simulink model "motorload"  (R2014b)
settings: Solver=ode23tb  StartTime=0.0  StopTime=10  MaxStep=.0001  MinStep=0.00001  RelTol=1e-3
undefined symbols (not defined in the file): sigbuilder_block
libraries: powerlib x145, simulink x25, powerlib_extras x4, dsparch4 x2, powerlib_meascontrol x1
(part 2 of 2)

== system motorload/STAR1/DC1/Subsystem2/PV Boost Converter1 ==
  Diode : powerlib/Power Electronics/Diode  Ron=0.001  Lon=0  Vf=0.8  IC=0  UseSnubber=off  Rs=500  Cs=250e-9  Measurements=on
  Mosfet : powerlib/Power Electronics/Mosfet  Ron=0.1  Lon=0  Rd=0.01  Vfd=0  IC=0  Rs=1e5  Cs=inf  Measurements=on
  PI CONTOLER : Subsystem
  Scope8 : Scope
      settings: YMin=66.25  YMax=66.75  SaveName=ScopeData4
  Series RLC Branch : powerlib/Elements/Series RLC Branch  LConnTagsString=__new0  RConnTagsString=__new0  BranchType=L  Resistance=1  Inductance=1e-3  SetiL0=off  InitialCurrent=0  Capacitance=1e-6  Setx0=off  InitialVoltage=0  Measurements=None
  Series RLC Branch1 : powerlib/Elements/Series RLC Branch  LConnTagsString=__new0  RConnTagsString=__new0  BranchType=C  Resistance=1  Inductance=12e-3  SetiL0=off  InitialCurrent=0  Capacitance=1000e-6  Setx0=off  InitialVoltage=0  Measurements=None
  Voltage Measurement1 : powerlib/Measurements/Voltage Measurement  PhasorSimulation=off  OutputType=Complex  PSBequivalent=0
  + : PMIOPort  Port=1  Side=Right
  - : PMIOPort  Port=2  Side=Right
  Vpv+ : PMIOPort  Tag=PMCPort  Port=3  Side=Left
  Vpv- : PMIOPort  Tag=PMCPort  Port=4  Side=Left
  wires:
  [G] -> Mosfet/1
  PI CONTOLER/1(Out1) -> [G]
  [A1] -> PI CONTOLER/1(In1)
  Voltage Measurement1/1 -> [A1], Scope8/1
  connections:
  Series RLC Branch/RConn1 -- Mosfet/LConn1 -- Diode/LConn1
  Mosfet/RConn1 -- Vpv-/RConn1 -- Series RLC Branch1/RConn1 -- -/RConn1 -- Voltage Measurement1/LConn2
  Vpv+/RConn1 -- Series RLC Branch/LConn1
  Series RLC Branch1/LConn1 -- Diode/RConn1 -- +/RConn1 -- Voltage Measurement1/LConn1

== system motorload/STAR1/DC1/Subsystem3/PV Boost Converter1 ==
  Diode : powerlib/Power Electronics/Diode  Ron=0.001  Lon=0  Vf=0.8  IC=0  UseSnubber=off  Rs=500  Cs=250e-9  Measurements=on
  Mosfet : powerlib/Power Electronics/Mosfet  Ron=0.1  Lon=0  Rd=0.01  Vfd=0  IC=0  Rs=1e5  Cs=inf  Measurements=on
  PI CONTOLER : Subsystem
  Scope8 : Scope
      settings: YMin=66.25  YMax=66.75  SaveName=ScopeData4
  Series RLC Branch : powerlib/Elements/Series RLC Branch  LConnTagsString=__new0  RConnTagsString=__new0  BranchType=L  Resistance=1  Inductance=1e-3  SetiL0=off  InitialCurrent=0  Capacitance=1e-6  Setx0=off  InitialVoltage=0  Measurements=None
  Series RLC Branch1 : powerlib/Elements/Series RLC Branch  LConnTagsString=__new0  RConnTagsString=__new0  BranchType=C  Resistance=1  Inductance=12e-3  SetiL0=off  InitialCurrent=0  Capacitance=1000e-6  Setx0=off  InitialVoltage=0  Measurements=None
  Voltage Measurement1 : powerlib/Measurements/Voltage Measurement  PhasorSimulation=off  OutputType=Complex  PSBequivalent=0
  + : PMIOPort  Port=1  Side=Right
  - : PMIOPort  Port=2  Side=Right
  Vpv+ : PMIOPort  Tag=PMCPort  Port=3  Side=Left
  Vpv- : PMIOPort  Tag=PMCPort  Port=4  Side=Left
  wires:
  [G] -> Mosfet/1
  PI CONTOLER/1(Out1) -> [G]
  [A1] -> PI CONTOLER/1(In1)
  Voltage Measurement1/1 -> [A1], Scope8/1
  connections:
  Series RLC Branch/RConn1 -- Mosfet/LConn1 -- Diode/LConn1
  Mosfet/RConn1 -- Vpv-/RConn1 -- Series RLC Branch1/RConn1 -- -/RConn1 -- Voltage Measurement1/LConn2
  Vpv+/RConn1 -- Series RLC Branch/LConn1
  Series RLC Branch1/LConn1 -- Diode/RConn1 -- +/RConn1 -- Voltage Measurement1/LConn1

== system motorload/STAR1/DC1/Subsystem4/PV Boost Converter1 ==
  Diode : powerlib/Power Electronics/Diode  Ron=0.001  Lon=0  Vf=0.8  IC=0  UseSnubber=off  Rs=500  Cs=250e-9  Measurements=on
  Mosfet : powerlib/Power Electronics/Mosfet  Ron=0.1  Lon=0  Rd=0.01  Vfd=0  IC=0  Rs=1e5  Cs=inf  Measurements=on
  PI CONTOLER : Subsystem
  Scope8 : Scope
      settings: YMin=66.25  YMax=66.75  SaveName=ScopeData4
  Series RLC Branch : powerlib/Elements/Series RLC Branch  LConnTagsString=__new0  RConnTagsString=__new0  BranchType=L  Resistance=1  Inductance=1e-3  SetiL0=off  InitialCurrent=0  Capacitance=1e-6  Setx0=off  InitialVoltage=0  Measurements=None
  Series RLC Branch1 : powerlib/Elements/Series RLC Branch  LConnTagsString=__new0  RConnTagsString=__new0  BranchType=C  Resistance=1  Inductance=12e-3  SetiL0=off  InitialCurrent=0  Capacitance=1000e-6  Setx0=off  InitialVoltage=0  Measurements=None
  Voltage Measurement1 : powerlib/Measurements/Voltage Measurement  PhasorSimulation=off  OutputType=Complex  PSBequivalent=0
  + : PMIOPort  Port=1  Side=Right
  - : PMIOPort  Port=2  Side=Right
  Vpv+ : PMIOPort  Tag=PMCPort  Port=3  Side=Left
  Vpv- : PMIOPort  Tag=PMCPort  Port=4  Side=Left
  wires:
  Voltage Measurement1/1 -> Scope8/1, [A1]
  [A1] -> PI CONTOLER/1(In1)
  PI CONTOLER/1(Out1) -> [G]
  [G] -> Mosfet/1
  connections:
  Voltage Measurement1/LConn1 -- +/RConn1 -- Diode/RConn1 -- Series RLC Branch1/LConn1
  Vpv+/RConn1 -- Series RLC Branch/LConn1
  Voltage Measurement1/LConn2 -- -/RConn1 -- Series RLC Branch1/RConn1 -- Vpv-/RConn1 -- Mosfet/RConn1
  Diode/LConn1 -- Mosfet/LConn1 -- Series RLC Branch/RConn1

== system motorload/STAR1/DC1/Subsystem6/PV Boost Converter1 ==
  Diode : powerlib/Power Electronics/Diode  Ron=0.001  Lon=0  Vf=0.8  IC=0  UseSnubber=off  Rs=500  Cs=250e-9  Measurements=on
  Mosfet : powerlib/Power Electronics/Mosfet  Ron=0.1  Lon=0  Rd=0.01  Vfd=0  IC=0  Rs=1e5  Cs=inf  Measurements=on
  PI CONTOLER : Subsystem
  Scope8 : Scope
      settings: YMin=66.25  YMax=66.75  SaveName=ScopeData4
  Series RLC Branch : powerlib/Elements/Series RLC Branch  LConnTagsString=__new0  RConnTagsString=__new0  BranchType=L  Resistance=1  Inductance=1e-3  SetiL0=off  InitialCurrent=0  Capacitance=1e-6  Setx0=off  InitialVoltage=0  Measurements=None
  Series RLC Branch1 : powerlib/Elements/Series RLC Branch  LConnTagsString=__new0  RConnTagsString=__new0  BranchType=C  Resistance=1  Inductance=12e-3  SetiL0=off  InitialCurrent=0  Capacitance=1000e-6  Setx0=off  InitialVoltage=0  Measurements=None
  Voltage Measurement1 : powerlib/Measurements/Voltage Measurement  PhasorSimulation=off  OutputType=Complex  PSBequivalent=0
  + : PMIOPort  Port=1  Side=Right
  - : PMIOPort  Port=2  Side=Right
  Vpv+ : PMIOPort  Tag=PMCPort  Port=3  Side=Left
  Vpv- : PMIOPort  Tag=PMCPort  Port=4  Side=Left
  wires:
  [G] -> Mosfet/1
  PI CONTOLER/1(Out1) -> [G]
  [A1] -> PI CONTOLER/1(In1)
  Voltage Measurement1/1 -> [A1], Scope8/1
  connections:
  Series RLC Branch/RConn1 -- Mosfet/LConn1 -- Diode/LConn1
  Mosfet/RConn1 -- Vpv-/RConn1 -- Series RLC Branch1/RConn1 -- -/RConn1 -- Voltage Measurement1/LConn2
  Vpv+/RConn1 -- Series RLC Branch/LConn1
  Series RLC Branch1/LConn1 -- Diode/RConn1 -- +/RConn1 -- Voltage Measurement1/LConn1

== system motorload/STAR1/DC2/Subsystem1/PV Boost Converter1 ==
  Diode : powerlib/Power Electronics/Diode  Ron=0.001  Lon=0  Vf=0.8  IC=0  UseSnubber=off  Rs=500  Cs=250e-9  Measurements=on
  Mosfet : powerlib/Power Electronics/Mosfet  Ron=0.1  Lon=0  Rd=0.01  Vfd=0  IC=0  Rs=1e5  Cs=inf  Measurements=on
  PI CONTOLER : Subsystem
  Scope8 : Scope
      settings: YMin=66.25  YMax=66.75  SaveName=ScopeData4
  Series RLC Branch : powerlib/Elements/Series RLC Branch  LConnTagsString=__new0  RConnTagsString=__new0  BranchType=L  Resistance=1  Inductance=1e-3  SetiL0=off  InitialCurrent=0  Capacitance=1e-6  Setx0=off  InitialVoltage=0  Measurements=None
  Series RLC Branch1 : powerlib/Elements/Series RLC Branch  LConnTagsString=__new0  RConnTagsString=__new0  BranchType=C  Resistance=1  Inductance=12e-3  SetiL0=off  InitialCurrent=0  Capacitance=1000e-6  Setx0=off  InitialVoltage=0  Measurements=None
  Voltage Measurement1 : powerlib/Measurements/Voltage Measurement  PhasorSimulation=off  OutputType=Complex  PSBequivalent=0
  + : PMIOPort  Port=1  Side=Right
  - : PMIOPort  Port=2  Side=Right
  Vpv+ : PMIOPort  Tag=PMCPort  Port=3  Side=Left
  Vpv- : PMIOPort  Tag=PMCPort  Port=4  Side=Left
  wires:
  [G] -> Mosfet/1
  PI CONTOLER/1(Out1) -> [G]
  [A1] -> PI CONTOLER/1(In1)
  Voltage Measurement1/1 -> [A1], Scope8/1
  connections:
  Series RLC Branch/RConn1 -- Mosfet/LConn1 -- Diode/LConn1
  Mosfet/RConn1 -- Vpv-/RConn1 -- Series RLC Branch1/RConn1 -- -/RConn1 -- Voltage Measurement1/LConn2
  Vpv+/RConn1 -- Series RLC Branch/LConn1
  Series RLC Branch1/LConn1 -- Diode/RConn1 -- +/RConn1 -- Voltage Measurement1/LConn1

== system motorload/STAR1/DC2/Subsystem2/PV Boost Converter1 ==
  Diode : powerlib/Power Electronics/Diode  Ron=0.001  Lon=0  Vf=0.8  IC=0  UseSnubber=off  Rs=500  Cs=250e-9  Measurements=on
  Mosfet : powerlib/Power Electronics/Mosfet  Ron=0.1  Lon=0  Rd=0.01  Vfd=0  IC=0  Rs=1e5  Cs=inf  Measurements=on
  PI CONTOLER : Subsystem
  Scope8 : Scope
      settings: YMin=66.25  YMax=66.75  SaveName=ScopeData4
  Series RLC Branch : powerlib/Elements/Series RLC Branch  LConnTagsString=__new0  RConnTagsString=__new0  BranchType=L  Resistance=1  Inductance=1e-3  SetiL0=off  InitialCurrent=0  Capacitance=1e-6  Setx0=off  InitialVoltage=0  Measurements=None
  Series RLC Branch1 : powerlib/Elements/Series RLC Branch  LConnTagsString=__new0  RConnTagsString=__new0  BranchType=C  Resistance=1  Inductance=12e-3  SetiL0=off  InitialCurrent=0  Capacitance=1000e-6  Setx0=off  InitialVoltage=0  Measurements=None
  Voltage Measurement1 : powerlib/Measurements/Voltage Measurement  PhasorSimulation=off  OutputType=Complex  PSBequivalent=0
  + : PMIOPort  Port=1  Side=Right
  - : PMIOPort  Port=2  Side=Right
  Vpv+ : PMIOPort  Tag=PMCPort  Port=3  Side=Left
  Vpv- : PMIOPort  Tag=PMCPort  Port=4  Side=Left
  wires:
  Voltage Measurement1/1 -> Scope8/1, [A1]
  [A1] -> PI CONTOLER/1(In1)
  PI CONTOLER/1(Out1) -> [G]
  [G] -> Mosfet/1
  connections:
  Voltage Measurement1/LConn1 -- +/RConn1 -- Diode/RConn1 -- Series RLC Branch1/LConn1
  Vpv+/RConn1 -- Series RLC Branch/LConn1
  Voltage Measurement1/LConn2 -- -/RConn1 -- Series RLC Branch1/RConn1 -- Vpv-/RConn1 -- Mosfet/RConn1
  Diode/LConn1 -- Mosfet/LConn1 -- Series RLC Branch/RConn1

== system motorload/STAR1/DC2/Subsystem3/PV Boost Converter1 ==
  Diode : powerlib/Power Electronics/Diode  Ron=0.001  Lon=0  Vf=0.8  IC=0  UseSnubber=off  Rs=500  Cs=250e-9  Measurements=on
  Mosfet : powerlib/Power Electronics/Mosfet  Ron=0.1  Lon=0  Rd=0.01  Vfd=0  IC=0  Rs=1e5  Cs=inf  Measurements=on
  PI CONTOLER : Subsystem
  Scope8 : Scope
      settings: YMin=66.25  YMax=66.75  SaveName=ScopeData4
  Series RLC Branch : powerlib/Elements/Series RLC Branch  LConnTagsString=__new0  RConnTagsString=__new0  BranchType=L  Resistance=1  Inductance=1e-3  SetiL0=off  InitialCurrent=0  Capacitance=1e-6  Setx0=off  InitialVoltage=0  Measurements=None
  Series RLC Branch1 : powerlib/Elements/Series RLC Branch  LConnTagsString=__new0  RConnTagsString=__new0  BranchType=C  Resistance=1  Inductance=12e-3  SetiL0=off  InitialCurrent=0  Capacitance=1000e-6  Setx0=off  InitialVoltage=0  Measurements=None
  Voltage Measurement1 : powerlib/Measurements/Voltage Measurement  PhasorSimulation=off  OutputType=Complex  PSBequivalent=0
  + : PMIOPort  Port=1  Side=Right
  - : PMIOPort  Port=2  Side=Right
  Vpv+ : PMIOPort  Tag=PMCPort  Port=3  Side=Left
  Vpv- : PMIOPort  Tag=PMCPort  Port=4  Side=Left
  wires:
  Voltage Measurement1/1 -> Scope8/1, [A1]
  [A1] -> PI CONTOLER/1(In1)
  PI CONTOLER/1(Out1) -> [G]
  [G] -> Mosfet/1
  connections:
  Voltage Measurement1/LConn1 -- +/RConn1 -- Diode/RConn1 -- Series RLC Branch1/LConn1
  Vpv+/RConn1 -- Series RLC Branch/LConn1
  Voltage Measurement1/LConn2 -- -/RConn1 -- Series RLC Branch1/RConn1 -- Vpv-/RConn1 -- Mosfet/RConn1
  Diode/LConn1 -- Mosfet/LConn1 -- Series RLC Branch/RConn1

== system motorload/STAR1/DC2/Subsystem4/PV Boost Converter1 ==
  Diode : powerlib/Power Electronics/Diode  Ron=0.001  Lon=0  Vf=0.8  IC=0  UseSnubber=off  Rs=500  Cs=250e-9  Measurements=on
  Mosfet : powerlib/Power Electronics/Mosfet  Ron=0.1  Lon=0  Rd=0.01  Vfd=0  IC=0  Rs=1e5  Cs=inf  Measurements=on
  PI CONTOLER : Subsystem
  Scope8 : Scope
      settings: YMin=66.25  YMax=66.75  SaveName=ScopeData4
  Series RLC Branch : powerlib/Elements/Series RLC Branch  LConnTagsString=__new0  RConnTagsString=__new0  BranchType=L  Resistance=1  Inductance=1e-3  SetiL0=off  InitialCurrent=0  Capacitance=1e-6  Setx0=off  InitialVoltage=0  Measurements=None
  Series RLC Branch1 : powerlib/Elements/Series RLC Branch  LConnTagsString=__new0  RConnTagsString=__new0  BranchType=C  Resistance=1  Inductance=12e-3  SetiL0=off  InitialCurrent=0  Capacitance=1000e-6  Setx0=off  InitialVoltage=0  Measurements=None
  Voltage Measurement1 : powerlib/Measurements/Voltage Measurement  PhasorSimulation=off  OutputType=Complex  PSBequivalent=0
  + : PMIOPort  Port=1  Side=Right
  - : PMIOPort  Port=2  Side=Right
  Vpv+ : PMIOPort  Tag=PMCPort  Port=3  Side=Left
  Vpv- : PMIOPort  Tag=PMCPort  Port=4  Side=Left
  wires:
  [G] -> Mosfet/1
  PI CONTOLER/1(Out1) -> [G]
  [A1] -> PI CONTOLER/1(In1)
  Voltage Measurement1/1 -> [A1], Scope8/1
  connections:
  Series RLC Branch/RConn1 -- Mosfet/LConn1 -- Diode/LConn1
  Mosfet/RConn1 -- Vpv-/RConn1 -- Series RLC Branch1/RConn1 -- -/RConn1 -- Voltage Measurement1/LConn2
  Vpv+/RConn1 -- Series RLC Branch/LConn1
  Series RLC Branch1/LConn1 -- Diode/RConn1 -- +/RConn1 -- Voltage Measurement1/LConn1

== system motorload/STAR1/DC2/Subsystem6/PV Boost Converter1 ==
  Diode : powerlib/Power Electronics/Diode  Ron=0.001  Lon=0  Vf=0.8  IC=0  UseSnubber=off  Rs=500  Cs=250e-9  Measurements=on
  Mosfet : powerlib/Power Electronics/Mosfet  Ron=0.1  Lon=0  Rd=0.01  Vfd=0  IC=0  Rs=1e5  Cs=inf  Measurements=on
  PI CONTOLER : Subsystem
  Scope8 : Scope
      settings: YMin=66.25  YMax=66.75  SaveName=ScopeData4
  Series RLC Branch : powerlib/Elements/Series RLC Branch  LConnTagsString=__new0  RConnTagsString=__new0  BranchType=L  Resistance=1  Inductance=1e-3  SetiL0=off  InitialCurrent=0  Capacitance=1e-6  Setx0=off  InitialVoltage=0  Measurements=None
  Series RLC Branch1 : powerlib/Elements/Series RLC Branch  LConnTagsString=__new0  RConnTagsString=__new0  BranchType=C  Resistance=1  Inductance=12e-3  SetiL0=off  InitialCurrent=0  Capacitance=1000e-6  Setx0=off  InitialVoltage=0  Measurements=None
  Voltage Measurement1 : powerlib/Measurements/Voltage Measurement  PhasorSimulation=off  OutputType=Complex  PSBequivalent=0
  + : PMIOPort  Port=1  Side=Right
  - : PMIOPort  Port=2  Side=Right
  Vpv+ : PMIOPort  Tag=PMCPort  Port=3  Side=Left
  Vpv- : PMIOPort  Tag=PMCPort  Port=4  Side=Left
  wires:
  Voltage Measurement1/1 -> Scope8/1, [A1]
  [A1] -> PI CONTOLER/1(In1)
  PI CONTOLER/1(Out1) -> [G]
  [G] -> Mosfet/1
  connections:
  Voltage Measurement1/LConn1 -- +/RConn1 -- Diode/RConn1 -- Series RLC Branch1/LConn1
  Vpv+/RConn1 -- Series RLC Branch/LConn1
  Voltage Measurement1/LConn2 -- -/RConn1 -- Series RLC Branch1/RConn1 -- Vpv-/RConn1 -- Mosfet/RConn1
  Diode/LConn1 -- Mosfet/LConn1 -- Series RLC Branch/RConn1

== system motorload/STAR1/PULSE/LOOKUP TABLE/If Action Subsystem ==
  In1 : Inport
  Action Port : ActionPort  ActionType=case
  Out1 : Outport
  wires:
  In1/1 -> Out1/1

== system motorload/STAR1/PULSE/LOOKUP TABLE/If Action Subsystem1 ==
  In1 : Inport
  Action Port : ActionPort  ActionType=case
  Out1 : Outport
  wires:
  In1/1 -> Out1/1

== system motorload/STAR1/PULSE/LOOKUP TABLE/If Action Subsystem10 ==
  In1 : Inport
  Action Port : ActionPort  ActionType=case
  Out1 : Outport
  wires:
  In1/1 -> Out1/1

== system motorload/STAR1/PULSE/LOOKUP TABLE/If Action Subsystem2 ==
  In1 : Inport
  Action Port : ActionPort  ActionType=case
  Out1 : Outport
  wires:
  In1/1 -> Out1/1

== system motorload/STAR1/PULSE/LOOKUP TABLE/If Action Subsystem3 ==
  In1 : Inport
  Action Port : ActionPort  ActionType=case
  Out1 : Outport
  wires:
  In1/1 -> Out1/1

== system motorload/STAR1/PULSE/LOOKUP TABLE/If Action Subsystem4 ==
  In1 : Inport
  Action Port : ActionPort  ActionType=case
  Out1 : Outport
  wires:
  In1/1 -> Out1/1

== system motorload/STAR1/PULSE/LOOKUP TABLE/If Action Subsystem5 ==
  In1 : Inport
  Action Port : ActionPort  ActionType=case
  Out1 : Outport
  wires:
  In1/1 -> Out1/1

== system motorload/STAR1/PULSE/LOOKUP TABLE/If Action Subsystem6 ==
  In1 : Inport
  Action Port : ActionPort  ActionType=case
  Out1 : Outport
  wires:
  In1/1 -> Out1/1

== system motorload/STAR1/PULSE/LOOKUP TABLE/If Action Subsystem7 ==
  In1 : Inport
  Action Port : ActionPort  ActionType=case
  Out1 : Outport
  wires:
  In1/1 -> Out1/1

== system motorload/STAR1/PULSE/LOOKUP TABLE/If Action Subsystem8 ==
  In1 : Inport
  Action Port : ActionPort  ActionType=case
  Out1 : Outport
  wires:
  In1/1 -> Out1/1

== system motorload/STAR1/PULSE/LOOKUP TABLE/If Action Subsystem9 ==
  In1 : Inport
  Action Port : ActionPort  ActionType=case
  Out1 : Outport
  wires:
  In1/1 -> Out1/1

== system motorload/STAR1/PULSE/LOOKUP TABLE1/If Action Subsystem ==
  In1 : Inport
  Action Port : ActionPort  ActionType=case
  Out1 : Outport
  wires:
  In1/1 -> Out1/1

== system motorload/STAR1/PULSE/LOOKUP TABLE1/If Action Subsystem1 ==
  In1 : Inport
  Action Port : ActionPort  ActionType=case
  Out1 : Outport
  wires:
  In1/1 -> Out1/1

== system motorload/STAR1/PULSE/LOOKUP TABLE1/If Action Subsystem10 ==
  In1 : Inport
  Action Port : ActionPort  ActionType=case
  Out1 : Outport
  wires:
  In1/1 -> Out1/1

== system motorload/STAR1/PULSE/LOOKUP TABLE1/If Action Subsystem2 ==
  In1 : Inport
  Action Port : ActionPort  ActionType=case
  Out1 : Outport
  wires:
  In1/1 -> Out1/1

== system motorload/STAR1/PULSE/LOOKUP TABLE1/If Action Subsystem3 ==
  In1 : Inport
  Action Port : ActionPort  ActionType=case
  Out1 : Outport
  wires:
  In1/1 -> Out1/1

== system motorload/STAR1/PULSE/LOOKUP TABLE1/If Action Subsystem4 ==
  In1 : Inport
  Action Port : ActionPort  ActionType=case
  Out1 : Outport
  wires:
  In1/1 -> Out1/1

== system motorload/STAR1/PULSE/LOOKUP TABLE1/If Action Subsystem5 ==
  In1 : Inport
  Action Port : ActionPort  ActionType=case
  Out1 : Outport
  wires:
  In1/1 -> Out1/1

== system motorload/STAR1/PULSE/LOOKUP TABLE1/If Action Subsystem6 ==
  In1 : Inport
  Action Port : ActionPort  ActionType=case
  Out1 : Outport
  wires:
  In1/1 -> Out1/1

== system motorload/STAR1/PULSE/LOOKUP TABLE1/If Action Subsystem7 ==
  In1 : Inport
  Action Port : ActionPort  ActionType=case
  Out1 : Outport
  wires:
  In1/1 -> Out1/1

== system motorload/STAR1/PULSE/LOOKUP TABLE1/If Action Subsystem8 ==
  In1 : Inport
  Action Port : ActionPort  ActionType=case
  Out1 : Outport
  wires:
  In1/1 -> Out1/1

== system motorload/STAR1/PULSE/LOOKUP TABLE1/If Action Subsystem9 ==
  In1 : Inport
  Action Port : ActionPort  ActionType=case
  Out1 : Outport
  wires:
  In1/1 -> Out1/1

== system motorload/STAR1/PULSE/LOOKUP TABLE2/If Action Subsystem ==
  In1 : Inport
  Action Port : ActionPort  ActionType=case
  Out1 : Outport
  wires:
  In1/1 -> Out1/1

== system motorload/STAR1/PULSE/LOOKUP TABLE2/If Action Subsystem1 ==
  In1 : Inport
  Action Port : ActionPort  ActionType=case
  Out1 : Outport
  wires:
  In1/1 -> Out1/1

== system motorload/STAR1/PULSE/LOOKUP TABLE2/If Action Subsystem10 ==
  In1 : Inport
  Action Port : ActionPort  ActionType=case
  Out1 : Outport
  wires:
  In1/1 -> Out1/1

== system motorload/STAR1/PULSE/LOOKUP TABLE2/If Action Subsystem2 ==
  In1 : Inport
  Action Port : ActionPort  ActionType=case
  Out1 : Outport
  wires:
  In1/1 -> Out1/1

== system motorload/STAR1/PULSE/LOOKUP TABLE2/If Action Subsystem3 ==
  In1 : Inport
  Action Port : ActionPort  ActionType=case
  Out1 : Outport
  wires:
  In1/1 -> Out1/1

== system motorload/STAR1/PULSE/LOOKUP TABLE2/If Action Subsystem4 ==
  In1 : Inport
  Action Port : ActionPort  ActionType=case
  Out1 : Outport
  wires:
  In1/1 -> Out1/1

== system motorload/STAR1/PULSE/LOOKUP TABLE2/If Action Subsystem5 ==
  In1 : Inport
  Action Port : ActionPort  ActionType=case
  Out1 : Outport
  wires:
  In1/1 -> Out1/1

== system motorload/STAR1/PULSE/LOOKUP TABLE2/If Action Subsystem6 ==
  In1 : Inport
  Action Port : ActionPort  ActionType=case
  Out1 : Outport
  wires:
  In1/1 -> Out1/1

== system motorload/STAR1/PULSE/LOOKUP TABLE2/If Action Subsystem7 ==
  In1 : Inport
  Action Port : ActionPort  ActionType=case
  Out1 : Outport
  wires:
  In1/1 -> Out1/1

== system motorload/STAR1/PULSE/LOOKUP TABLE2/If Action Subsystem8 ==
  In1 : Inport
  Action Port : ActionPort  ActionType=case
  Out1 : Outport
  wires:
  In1/1 -> Out1/1

== system motorload/STAR1/PULSE/LOOKUP TABLE2/If Action Subsystem9 ==
  In1 : Inport
  Action Port : ActionPort  ActionType=case
  Out1 : Outport
  wires:
  In1/1 -> Out1/1

== system motorload/STAR1/PULSE/R1/Signal Builder ==
  Demux : Demux  Tag=STV Demux  Outputs=1
  FromWs : FromWorkspace  Tag=STV FromWs  VariableName=tuvar  SampleTime=0
      SigBuilderData=|
      | common.afterFinalStr = 'Extrapolate'
      | common.sampleTime = 0
      | dataSet.timeRange = [0 10]
      | dataSet.name = 'Group 1'
      | sbobj.Groups.Name = 'Group 1'
      | sbobj.Groups.Signals.Name = 'Signal 1'
      | sbobj.Groups.Signals.XData = [0 0.98 0.98 1.98 1.98 2.96 2.96 3.96 3.96 5 5 6 6 7 7 8 8 9 9 10]
      | sbobj.Groups.Signals.YData = [0.2 0.2 0.4 0.4 0.6 0.6 0.8 0.8 1 1 1.2 1.2 1.4 1.4 1.6 1.6 1.8 1.8 2 2]
  Signal 1 : Outport  Tag=STV Outport
  wires:
  Demux/1 -> Signal 1/1
  FromWs/1 -> Demux/1

== system motorload/STAR1/DC/Subsystem1/PV Boost Converter1/PI CONTOLER ==
  In1 : Inport
  Add : Sum  Inputs=+-
  Constant1 : Constant  Value=66.5
  Gain1 : Gain  Gain=0.1
  Gain2 : Gain  Gain=5
  Integrator : Integrator
  Mux : Mux  Inputs=2
  Relational Operator1 : RelationalOperator  OutDataTypeStr=boolean
  Repeating Sequence : simulink/Sources/Repeating Sequence  rep_seq_t=[0 0.0001 0.0002]  rep_seq_y=[0 10 0]
  Saturation1 : Saturate  UpperLimit=10  LowerLimit=0
  Scope4 : Scope
      settings: SaveName=ScopeData9
  Sum : Sum  Inputs=|++
  Out1 : Outport
  wires:
  In1/1 -> Add/2, Mux/2
  Constant1/1 -> Mux/1, Add/1
  Add/1 -> Gain1/1, Gain2/1
  Repeating Sequence/1 -> Relational Operator1/1
  Relational Operator1/1 -> Out1/1
  Gain1/1 -> Sum/1
  Integrator/1 -> Sum/2
  Mux/1 -> Scope4/1
  Sum/1 -> Saturation1/1
  Gain2/1 -> Integrator/1
  Saturation1/1 -> Relational Operator1/2

== system motorload/STAR1/DC/Subsystem2/PV Boost Converter1/PI CONTOLER ==
  In1 : Inport
  Add : Sum  Inputs=+-
  Constant1 : Constant  Value=66.5
  Gain1 : Gain  Gain=0.1
  Gain2 : Gain  Gain=5
  Integrator : Integrator
  Mux : Mux  Inputs=2
  Relational Operator1 : RelationalOperator  OutDataTypeStr=boolean
  Repeating Sequence : simulink/Sources/Repeating Sequence  rep_seq_t=[0 0.0001 0.0002]  rep_seq_y=[0 10 0]
  Saturation1 : Saturate  UpperLimit=10  LowerLimit=0
  Scope4 : Scope
      settings: SaveName=ScopeData9
  Sum : Sum  Inputs=|++
  Out1 : Outport
  wires:
  Saturation1/1 -> Relational Operator1/2
  Gain2/1 -> Integrator/1
  Sum/1 -> Saturation1/1
  Mux/1 -> Scope4/1
  Integrator/1 -> Sum/2
  Gain1/1 -> Sum/1
  Relational Operator1/1 -> Out1/1
  Repeating Sequence/1 -> Relational Operator1/1
  Add/1 -> Gain2/1, Gain1/1
  Constant1/1 -> Add/1, Mux/1
  In1/1 -> Mux/2, Add/2

== system motorload/STAR1/DC/Subsystem3/PV Boost Converter1/PI CONTOLER ==
  In1 : Inport
  Add : Sum  Inputs=+-
  Constant1 : Constant  Value=66.5
  Gain1 : Gain  Gain=0.1
  Gain2 : Gain  Gain=5
  Integrator : Integrator
  Mux : Mux  Inputs=2
  Relational Operator1 : RelationalOperator  OutDataTypeStr=boolean
  Repeating Sequence : simulink/Sources/Repeating Sequence  rep_seq_t=[0 0.0001 0.0002]  rep_seq_y=[0 10 0]
  Saturation1 : Saturate  UpperLimit=10  LowerLimit=0
  Scope4 : Scope
      settings: SaveName=ScopeData9
  Sum : Sum  Inputs=|++
  Out1 : Outport
  wires:
  Saturation1/1 -> Relational Operator1/2
  Gain2/1 -> Integrator/1
  Sum/1 -> Saturation1/1
  Mux/1 -> Scope4/1
  Integrator/1 -> Sum/2
  Gain1/1 -> Sum/1
  Relational Operator1/1 -> Out1/1
  Repeating Sequence/1 -> Relational Operator1/1
  Add/1 -> Gain2/1, Gain1/1
  Constant1/1 -> Add/1, Mux/1
  In1/1 -> Mux/2, Add/2

== system motorload/STAR1/DC/Subsystem4/PV Boost Converter1/PI CONTOLER ==
  In1 : Inport
  Add : Sum  Inputs=+-
  Constant1 : Constant  Value=66.5
  Gain1 : Gain  Gain=0.1
  Gain2 : Gain  Gain=5
  Integrator : Integrator
  Mux : Mux  Inputs=2
  Relational Operator1 : RelationalOperator  OutDataTypeStr=boolean
  Repeating Sequence : simulink/Sources/Repeating Sequence  rep_seq_t=[0 0.0001 0.0002]  rep_seq_y=[0 10 0]
  Saturation1 : Saturate  UpperLimit=10  LowerLimit=0
  Scope4 : Scope
      settings: SaveName=ScopeData9
  Sum : Sum  Inputs=|++
  Out1 : Outport
  wires:
  In1/1 -> Add/2, Mux/2
  Constant1/1 -> Mux/1, Add/1
  Add/1 -> Gain1/1, Gain2/1
  Repeating Sequence/1 -> Relational Operator1/1
  Relational Operator1/1 -> Out1/1
  Gain1/1 -> Sum/1
  Integrator/1 -> Sum/2
  Mux/1 -> Scope4/1
  Sum/1 -> Saturation1/1
  Gain2/1 -> Integrator/1
  Saturation1/1 -> Relational Operator1/2

== system motorload/STAR1/DC/Subsystem6/PV Boost Converter1/PI CONTOLER ==
  In1 : Inport
  Add : Sum  Inputs=+-
  Constant1 : Constant  Value=66.5
  Gain1 : Gain  Gain=0.1
  Gain2 : Gain  Gain=5
  Integrator : Integrator
  Mux : Mux  Inputs=2
  Relational Operator1 : RelationalOperator  OutDataTypeStr=boolean
  Repeating Sequence : simulink/Sources/Repeating Sequence  rep_seq_t=[0 0.0001 0.0002]  rep_seq_y=[0 10 0]
  Saturation1 : Saturate  UpperLimit=10  LowerLimit=0
  Scope4 : Scope
      settings: SaveName=ScopeData9
  Sum : Sum  Inputs=|++
  Out1 : Outport
  wires:
  Saturation1/1 -> Relational Operator1/2
  Gain2/1 -> Integrator/1
  Sum/1 -> Saturation1/1
  Mux/1 -> Scope4/1
  Integrator/1 -> Sum/2
  Gain1/1 -> Sum/1
  Relational Operator1/1 -> Out1/1
  Repeating Sequence/1 -> Relational Operator1/1
  Add/1 -> Gain2/1, Gain1/1
  Constant1/1 -> Add/1, Mux/1
  In1/1 -> Mux/2, Add/2

== system motorload/STAR1/DC1/Subsystem1/PV Boost Converter1/PI CONTOLER ==
  In1 : Inport
  Add : Sum  Inputs=+-
  Constant1 : Constant  Value=66.5
  Gain1 : Gain  Gain=0.1
  Gain2 : Gain  Gain=5
  Integrator : Integrator
  Mux : Mux  Inputs=2
  Relational Operator1 : RelationalOperator  OutDataTypeStr=boolean
  Repeating Sequence : simulink/Sources/Repeating Sequence  rep_seq_t=[0 0.0001 0.0002]  rep_seq_y=[0 10 0]
  Saturation1 : Saturate  UpperLimit=10  LowerLimit=0
  Scope4 : Scope
      settings: SaveName=ScopeData9
  Sum : Sum  Inputs=|++
  Out1 : Outport
  wires:
  Saturation1/1 -> Relational Operator1/2
  Gain2/1 -> Integrator/1
  Sum/1 -> Saturation1/1
  Mux/1 -> Scope4/1
  Integrator/1 -> Sum/2
  Gain1/1 -> Sum/1
  Relational Operator1/1 -> Out1/1
  Repeating Sequence/1 -> Relational Operator1/1
  Add/1 -> Gain2/1, Gain1/1
  Constant1/1 -> Add/1, Mux/1
  In1/1 -> Mux/2, Add/2

== system motorload/STAR1/DC1/Subsystem2/PV Boost Converter1/PI CONTOLER ==
  In1 : Inport
  Add : Sum  Inputs=+-
  Constant1 : Constant  Value=66.5
  Gain1 : Gain  Gain=0.1
  Gain2 : Gain  Gain=5
  Integrator : Integrator
  Mux : Mux  Inputs=2
  Relational Operator1 : RelationalOperator  OutDataTypeStr=boolean
  Repeating Sequence : simulink/Sources/Repeating Sequence  rep_seq_t=[0 0.0001 0.0002]  rep_seq_y=[0 10 0]
  Saturation1 : Saturate  UpperLimit=10  LowerLimit=0
  Scope4 : Scope
      settings: SaveName=ScopeData9
  Sum : Sum  Inputs=|++
  Out1 : Outport
  wires:
  In1/1 -> Add/2, Mux/2
  Constant1/1 -> Mux/1, Add/1
  Add/1 -> Gain1/1, Gain2/1
  Repeating Sequence/1 -> Relational Operator1/1
  Relational Operator1/1 -> Out1/1
  Gain1/1 -> Sum/1
  Integrator/1 -> Sum/2
  Mux/1 -> Scope4/1
  Sum/1 -> Saturation1/1
  Gain2/1 -> Integrator/1
  Saturation1/1 -> Relational Operator1/2

== system motorload/STAR1/DC1/Subsystem3/PV Boost Converter1/PI CONTOLER ==
  In1 : Inport
  Add : Sum  Inputs=+-
  Constant1 : Constant  Value=66.5
  Gain1 : Gain  Gain=0.1
  Gain2 : Gain  Gain=5
  Integrator : Integrator
  Mux : Mux  Inputs=2
  Relational Operator1 : RelationalOperator  OutDataTypeStr=boolean
  Repeating Sequence : simulink/Sources/Repeating Sequence  rep_seq_t=[0 0.0001 0.0002]  rep_seq_y=[0 10 0]
  Saturation1 : Saturate  UpperLimit=10  LowerLimit=0
  Scope4 : Scope
      settings: SaveName=ScopeData9
  Sum : Sum  Inputs=|++
  Out1 : Outport
  wires:
  In1/1 -> Add/2, Mux/2
  Constant1/1 -> Mux/1, Add/1
  Add/1 -> Gain1/1, Gain2/1
  Repeating Sequence/1 -> Relational Operator1/1
  Relational Operator1/1 -> Out1/1
  Gain1/1 -> Sum/1
  Integrator/1 -> Sum/2
  Mux/1 -> Scope4/1
  Sum/1 -> Saturation1/1
  Gain2/1 -> Integrator/1
  Saturation1/1 -> Relational Operator1/2

== system motorload/STAR1/DC1/Subsystem4/PV Boost Converter1/PI CONTOLER ==
  In1 : Inport
  Add : Sum  Inputs=+-
  Constant1 : Constant  Value=66.5
  Gain1 : Gain  Gain=0.1
  Gain2 : Gain  Gain=5
  Integrator : Integrator
  Mux : Mux  Inputs=2
  Relational Operator1 : RelationalOperator  OutDataTypeStr=boolean
  Repeating Sequence : simulink/Sources/Repeating Sequence  rep_seq_t=[0 0.0001 0.0002]  rep_seq_y=[0 10 0]
  Saturation1 : Saturate  UpperLimit=10  LowerLimit=0
  Scope4 : Scope
      settings: SaveName=ScopeData9
  Sum : Sum  Inputs=|++
  Out1 : Outport
  wires:
  Saturation1/1 -> Relational Operator1/2
  Gain2/1 -> Integrator/1
  Sum/1 -> Saturation1/1
  Mux/1 -> Scope4/1
  Integrator/1 -> Sum/2
  Gain1/1 -> Sum/1
  Relational Operator1/1 -> Out1/1
  Repeating Sequence/1 -> Relational Operator1/1
  Add/1 -> Gain2/1, Gain1/1
  Constant1/1 -> Add/1, Mux/1
  In1/1 -> Mux/2, Add/2

== system motorload/STAR1/DC1/Subsystem6/PV Boost Converter1/PI CONTOLER ==
  In1 : Inport
  Add : Sum  Inputs=+-
  Constant1 : Constant  Value=66.5
  Gain1 : Gain  Gain=0.1
  Gain2 : Gain  Gain=5
  Integrator : Integrator
  Mux : Mux  Inputs=2
  Relational Operator1 : RelationalOperator  OutDataTypeStr=boolean
  Repeating Sequence : simulink/Sources/Repeating Sequence  rep_seq_t=[0 0.0001 0.0002]  rep_seq_y=[0 10 0]
  Saturation1 : Saturate  UpperLimit=10  LowerLimit=0
  Scope4 : Scope
      settings: SaveName=ScopeData9
  Sum : Sum  Inputs=|++
  Out1 : Outport
  wires:
  In1/1 -> Add/2, Mux/2
  Constant1/1 -> Mux/1, Add/1
  Add/1 -> Gain1/1, Gain2/1
  Repeating Sequence/1 -> Relational Operator1/1
  Relational Operator1/1 -> Out1/1
  Gain1/1 -> Sum/1
  Integrator/1 -> Sum/2
  Mux/1 -> Scope4/1
  Sum/1 -> Saturation1/1
  Gain2/1 -> Integrator/1
  Saturation1/1 -> Relational Operator1/2

== system motorload/STAR1/DC2/Subsystem1/PV Boost Converter1/PI CONTOLER ==
  In1 : Inport
  Add : Sum  Inputs=+-
  Constant1 : Constant  Value=66.5
  Gain1 : Gain  Gain=0.1
  Gain2 : Gain  Gain=5
  Integrator : Integrator
  Mux : Mux  Inputs=2
  Relational Operator1 : RelationalOperator  OutDataTypeStr=boolean
  Repeating Sequence : simulink/Sources/Repeating Sequence  rep_seq_t=[0 0.0001 0.0002]  rep_seq_y=[0 10 0]
  Saturation1 : Saturate  UpperLimit=10  LowerLimit=0
  Scope4 : Scope
      settings: SaveName=ScopeData9
  Sum : Sum  Inputs=|++
  Out1 : Outport
  wires:
  In1/1 -> Add/2, Mux/2
  Constant1/1 -> Mux/1, Add/1
  Add/1 -> Gain1/1, Gain2/1
  Repeating Sequence/1 -> Relational Operator1/1
  Relational Operator1/1 -> Out1/1
  Gain1/1 -> Sum/1
  Integrator/1 -> Sum/2
  Mux/1 -> Scope4/1
  Sum/1 -> Saturation1/1
  Gain2/1 -> Integrator/1
  Saturation1/1 -> Relational Operator1/2

== system motorload/STAR1/DC2/Subsystem2/PV Boost Converter1/PI CONTOLER ==
  In1 : Inport
  Add : Sum  Inputs=+-
  Constant1 : Constant  Value=66.5
  Gain1 : Gain  Gain=0.1
  Gain2 : Gain  Gain=5
  Integrator : Integrator
  Mux : Mux  Inputs=2
  Relational Operator1 : RelationalOperator  OutDataTypeStr=boolean
  Repeating Sequence : simulink/Sources/Repeating Sequence  rep_seq_t=[0 0.0001 0.0002]  rep_seq_y=[0 10 0]
  Saturation1 : Saturate  UpperLimit=10  LowerLimit=0
  Scope4 : Scope
      settings: SaveName=ScopeData9
  Sum : Sum  Inputs=|++
  Out1 : Outport
  wires:
  Saturation1/1 -> Relational Operator1/2
  Gain2/1 -> Integrator/1
  Sum/1 -> Saturation1/1
  Mux/1 -> Scope4/1
  Integrator/1 -> Sum/2
  Gain1/1 -> Sum/1
  Relational Operator1/1 -> Out1/1
  Repeating Sequence/1 -> Relational Operator1/1
  Add/1 -> Gain2/1, Gain1/1
  Constant1/1 -> Add/1, Mux/1
  In1/1 -> Mux/2, Add/2

== system motorload/STAR1/DC2/Subsystem3/PV Boost Converter1/PI CONTOLER ==
  In1 : Inport
  Add : Sum  Inputs=+-
  Constant1 : Constant  Value=66.5
  Gain1 : Gain  Gain=0.1
  Gain2 : Gain  Gain=5
  Integrator : Integrator
  Mux : Mux  Inputs=2
  Relational Operator1 : RelationalOperator  OutDataTypeStr=boolean
  Repeating Sequence : simulink/Sources/Repeating Sequence  rep_seq_t=[0 0.0001 0.0002]  rep_seq_y=[0 10 0]
  Saturation1 : Saturate  UpperLimit=10  LowerLimit=0
  Scope4 : Scope
      settings: SaveName=ScopeData9
  Sum : Sum  Inputs=|++
  Out1 : Outport
  wires:
  Saturation1/1 -> Relational Operator1/2
  Gain2/1 -> Integrator/1
  Sum/1 -> Saturation1/1
  Mux/1 -> Scope4/1
  Integrator/1 -> Sum/2
  Gain1/1 -> Sum/1
  Relational Operator1/1 -> Out1/1
  Repeating Sequence/1 -> Relational Operator1/1
  Add/1 -> Gain2/1, Gain1/1
  Constant1/1 -> Add/1, Mux/1
  In1/1 -> Mux/2, Add/2

== system motorload/STAR1/DC2/Subsystem4/PV Boost Converter1/PI CONTOLER ==
  In1 : Inport
  Add : Sum  Inputs=+-
  Constant1 : Constant  Value=66.5
  Gain1 : Gain  Gain=0.1
  Gain2 : Gain  Gain=5
  Integrator : Integrator
  Mux : Mux  Inputs=2
  Relational Operator1 : RelationalOperator  OutDataTypeStr=boolean
  Repeating Sequence : simulink/Sources/Repeating Sequence  rep_seq_t=[0 0.0001 0.0002]  rep_seq_y=[0 10 0]
  Saturation1 : Saturate  UpperLimit=10  LowerLimit=0
  Scope4 : Scope
      settings: SaveName=ScopeData9
  Sum : Sum  Inputs=|++
  Out1 : Outport
  wires:
  In1/1 -> Add/2, Mux/2
  Constant1/1 -> Mux/1, Add/1
  Add/1 -> Gain1/1, Gain2/1
  Repeating Sequence/1 -> Relational Operator1/1
  Relational Operator1/1 -> Out1/1
  Gain1/1 -> Sum/1
  Integrator/1 -> Sum/2
  Mux/1 -> Scope4/1
  Sum/1 -> Saturation1/1
  Gain2/1 -> Integrator/1
  Saturation1/1 -> Relational Operator1/2

== system motorload/STAR1/DC2/Subsystem6/PV Boost Converter1/PI CONTOLER ==
  In1 : Inport
  Add : Sum  Inputs=+-
  Constant1 : Constant  Value=66.5
  Gain1 : Gain  Gain=0.1
  Gain2 : Gain  Gain=5
  Integrator : Integrator
  Mux : Mux  Inputs=2
  Relational Operator1 : RelationalOperator  OutDataTypeStr=boolean
  Repeating Sequence : simulink/Sources/Repeating Sequence  rep_seq_t=[0 0.0001 0.0002]  rep_seq_y=[0 10 0]
  Saturation1 : Saturate  UpperLimit=10  LowerLimit=0
  Scope4 : Scope
      settings: SaveName=ScopeData9
  Sum : Sum  Inputs=|++
  Out1 : Outport
  wires:
  Saturation1/1 -> Relational Operator1/2
  Gain2/1 -> Integrator/1
  Sum/1 -> Saturation1/1
  Mux/1 -> Scope4/1
  Integrator/1 -> Sum/2
  Gain1/1 -> Sum/1
  Relational Operator1/1 -> Out1/1
  Repeating Sequence/1 -> Relational Operator1/1
  Add/1 -> Gain2/1, Gain1/1
  Constant1/1 -> Add/1, Mux/1
  In1/1 -> Mux/2, Add/2
